simulink model "task_3_scheme"  (R2024a)
settings: Solver=FixedStepAuto  StartTime=0.0  StopTime=30.0  FixedStep=0.001  RelTol=1e-3
libraries: simulink x2
settings Model: Creator=alexe  LastModifiedBy=alexe

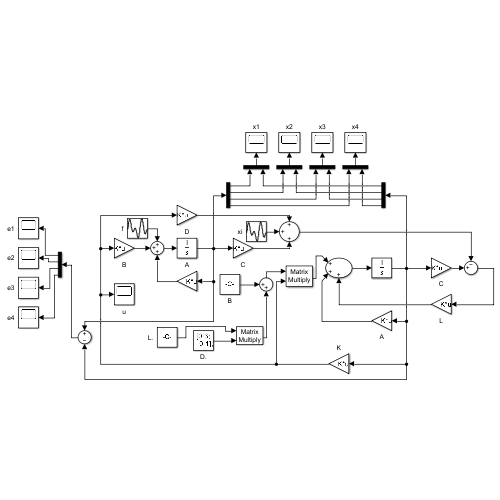
[thumbnail: Simulink's stored preview of the top-level diagram]
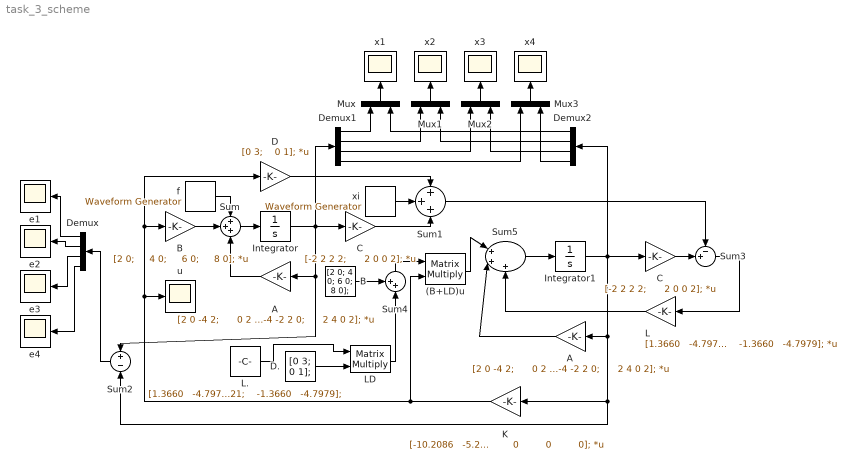
== system task_3_scheme ==
  (B+LD)u : Product  Multiplication=Matrix(*)
  A : Gain  Gain=|  Multiplication=Matrix(K*u)
      | [2 0 -4 2;
      |      0 2 -2 4;
      |     -4 -2 2 0;
      |      2 4 0 2];
  B : Gain  Gain=|  Multiplication=Matrix(K*u)
      | [2 0;
      |     4 0;
      |     6 0;
      |     8 0];
  C : Gain  Gain=|  Multiplication=Matrix(K*u)
      | [-2 2 2 2;
      |      2 0 0 2];
  D : Gain  Gain=|  Multiplication=Matrix(K*u)
      | [0 3;
      |    0 1];
  D. : Constant  Value=|  VectorParams1D=off
      | [0 3;
      |    0 1];
  Demux : Demux
  Demux1 : Demux
  Demux2 : Demux
  Integrator : Integrator  InitialCondition=[1;1;1;1]
  Integrator1 : Integrator  InitialCondition=[0; 0; 0; 0]
  K : Gain  Gain=|  Multiplication=Matrix(K*u)
      | [-10.2086   -5.2443    9.8924   -5.5605;
      |          0         0         0         0];
  L : Gain  Gain=|  Multiplication=Matrix(K*u)
      | [1.3660   -4.7979;
      |    -1.3660   -6.2121;
      |    -1.3660    6.2121;
      |    -1.3660   -4.7979];
  L. : Constant  Value=|  VectorParams1D=off
      | [1.3660   -4.7979;
      |    -1.3660   -6.2121;
      |    -1.3660    6.2121;
      |    -1.3660   -4.7979];
  LD : Product  Multiplication=Matrix(*)
  Mux{,1..3} (4 alike) : Mux  Inputs=2
  Sum : Sum  Inputs=+++
  Sum1 : Sum  Inputs=+++
  Sum2 : Sum  Inputs=+|-
  Sum3 : Sum  Inputs=-+|
  Sum4 : Sum  Inputs=++|
  Sum5 : Sum  Inputs=|+++
  e{1..4} (4 alike) : Scope
  f : simulink/Sources/Waveform Generator  OutMin=[]  OutMax=[]  OutDataTypeStr=double  SelectedSignal=1  Signals=sin('Amplitude',0.1,'Frequency',pi/3,'Phase',0)#sin('Amplitude',-0.3,'Frequency',pi/3,'Phase',pi/2)  BlockNames=MultiportSwitch_f74ed6b8ace6456#MultiportSwitch_4f882b6a03b0400  SampleTime=0.1
  u : Scope
  x{1..4} (4 alike) : Scope
  xi : simulink/Sources/Waveform Generator  OutMin=[]  OutMax=[]  OutDataTypeStr=double  SelectedSignal=1  Signals=sin('Amplitude',-0.5,'Frequency',pi/3,'Phase',0)#sin('Amplitude',0.2,'Frequency',pi/3,'Phase',pi/2)  BlockNames=MultiportSwitch_4b5f4914bd0a4c2#MultiportSwitch_51becfe54898412  SampleTime=0.1
  А : Gain  Gain=|  Multiplication=Matrix(K*u)
      | [2 0 -4 2;
      |      0 2 -2 4;
      |     -4 -2 2 0;
      |      2 4 0 2];
  В : Constant  Value=|  VectorParams1D=off
      | [2 0;
      |     4 0;
      |     6 0;
      |     8 0];
  С : Gain  Gain=|  Multiplication=Matrix(K*u)
      | [-2 2 2 2;
      |      2 0 0 2];
  wires:
  Sum/1 -> Integrator/1
  Integrator/1 -> C/1, Demux1/1, A/1, Sum2/1
  K/1 -> u/1, D/1, B/1, (B+LD)u/2
  Integrator1/1 -> Demux2/1, Sum2/2, K/1, А/1, С/1
  С/1 -> Sum3/2
  Sum1/1 -> Sum3/1
  Sum3/1 -> L/1
  L./1 -> LD/1
  D./1 -> LD/2
  В/1 -> Sum4/1
  LD/1 -> Sum4/2
  Sum4/1 -> (B+LD)u/1
  Sum5/1 -> Integrator1/1
  (B+LD)u/1 -> Sum5/1
  D/1 -> Sum1/1
  Sum2/1 -> Demux/1
  Demux/1 -> e1/1
  Demux/2 -> e2/1
  Demux/3 -> e3/1
  Demux/4 -> e4/1
  Demux1/1 -> Mux/1
  Demux2/1 -> Mux/2
  Mux/1 -> x1/1
  Demux1/2 -> Mux1/1
  Mux1/1 -> x2/1
  Demux2/2 -> Mux1/2
  Mux2/1 -> x3/1
  Mux3/1 -> x4/1
  Demux1/3 -> Mux2/1
  Demux2/3 -> Mux2/2
  Demux1/4 -> Mux3/1
  Demux2/4 -> Mux3/2
  A/1 -> Sum/3
  B/1 -> Sum/2
  f/1 -> Sum/1
  C/1 -> Sum1/3
  xi/1 -> Sum1/2
  А/1 -> Sum5/2
  L/1 -> Sum5/3
